simulink subsystem "SSD1306"  (R2024b)
settings: Solver=VariableStepAuto  StartTime=0.0  StopTime=10.0  RelTol=1e-3
settings Model: Creator=JesseJabezArendse  LastModifiedBy=JesseJabezArendse

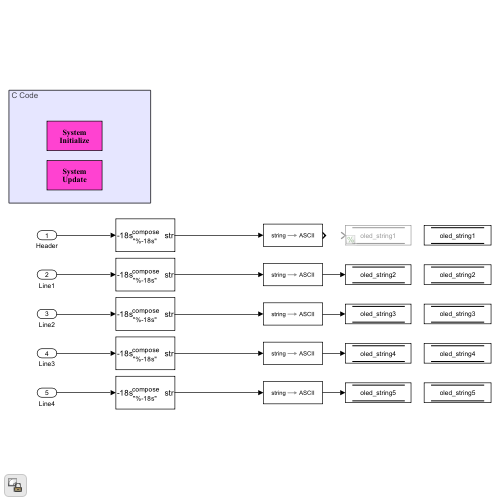
[thumbnail: Simulink's stored preview of the top-level diagram]
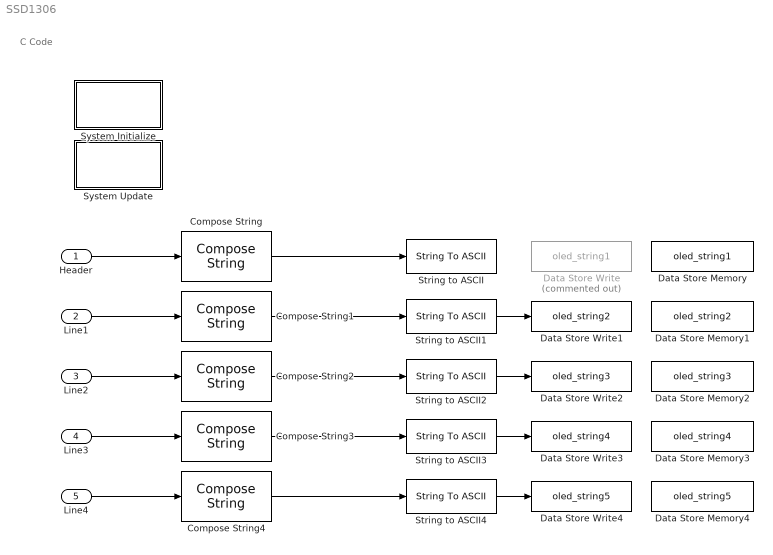
== system SSD1306 ==
  note: C Code
  Header : Inport
  Line1 : Inport  Port=2
  Line2 : Inport  Port=3
  Line3 : Inport  Port=4
  Line4 : Inport  Port=5
  Compose String{,1..4} (5 alike) : ComposeString  Format="\"%-18s\""
  Data Store Memory : DataStoreMemory  DataStoreName=oled_string1  WriteAfterWriteMsg=warning  ShowAdditionalParam=off  OutDataTypeStr=uint8  Dimensions=18
  Data Store Memory1 : DataStoreMemory  DataStoreName=oled_string2  WriteAfterWriteMsg=warning  ShowAdditionalParam=off  OutDataTypeStr=uint8  Dimensions=18
  Data Store Memory2 : DataStoreMemory  DataStoreName=oled_string3  WriteAfterWriteMsg=warning  ShowAdditionalParam=off  OutDataTypeStr=uint8  Dimensions=18
  Data Store Memory3 : DataStoreMemory  DataStoreName=oled_string4  WriteAfterWriteMsg=warning  ShowAdditionalParam=off  OutDataTypeStr=uint8  Dimensions=18
  Data Store Memory4 : DataStoreMemory  DataStoreName=oled_string5  WriteAfterWriteMsg=warning  ShowAdditionalParam=off  OutDataTypeStr=uint8  Dimensions=18
  Data Store Write : DataStoreWrite  Commented=on  DataStoreName=oled_string1  IndexOptions=Index vector (dialog)  Indices=1  OutputSizes=1
  Data Store Write1 : DataStoreWrite  DataStoreName=oled_string2  IndexOptions=Index vector (dialog)  Indices=1  OutputSizes=1
  Data Store Write2 : DataStoreWrite  DataStoreName=oled_string3  IndexOptions=Index vector (dialog)  Indices=1  OutputSizes=1
  Data Store Write3 : DataStoreWrite  DataStoreName=oled_string4  IndexOptions=Index vector (dialog)  Indices=1  OutputSizes=1
  Data Store Write4 : DataStoreWrite  DataStoreName=oled_string5  IndexOptions=Index vector (dialog)  Indices=1  OutputSizes=1
  String to ASCII{,1..4} (5 alike) : StringToASCII  OutputVectorSize=18
  System Initialize : Subsystem  mask(System Initialize){ShowInLibBrowser=0}
      mask prompts: ShowInLibBrowser "Simulink:masks:CustCodeMaskParam1_MP"
      settings: CopyFcn=cccopyfcn(gcb)  OpenFcn=ccopenfcn('System Initialize Function')
      mask Help: eval('feval(''rtwprivate'',''rtwhelpview'',''rtw_sys_initialize_block'')');
      mask Display: disp('System\nInitialize');
  System Update : Subsystem  mask(System Update){ShowInLibBrowser=0}
      mask prompts: ShowInLibBrowser "Simulink:masks:CustCodeMaskParam1_MP"
      settings: CopyFcn=cccopyfcn(gcb)  OpenFcn=ccopenfcn('System Update Function')
      mask Help: eval('feval(''rtwprivate'',''rtwhelpview'',''rtw_sys_update_block'')');
      mask Display: disp('System\nUpdate');
  wires:
  Header/1 -> Compose String/1
  String to ASCII1/1 -> Data Store Write1/1
  String to ASCII2/1 -> Data Store Write2/1
  Line1/1 -> Compose String1/1
  Line2/1 -> Compose String2/1
  Compose String/1 -> String to ASCII/1
  Compose String1/1 -> String to ASCII1/1
  Compose String2/1 -> String to ASCII2/1
  Compose String3/1 -> String to ASCII3/1
  Line3/1 -> Compose String3/1
  String to ASCII3/1 -> Data Store Write3/1
  Compose String4/1 -> String to ASCII4/1
  Line4/1 -> Compose String4/1
  String to ASCII4/1 -> Data Store Write4/1

== system SSD1306/System Initialize ==

== system SSD1306/System Update ==
